simulink model "sixDOF_SIM"  (R2015a)
settings: Solver=ode45  StartTime=0.0  StopTime=t_total  MaxStep=60  RelTol=1e-3
values from neighbouring files (symbols this model uses):
  A0 = zeros(3,3)    [PS2.m]    (also in PS3.m = getDCM(triad1, triad2); PS4.m = getDCM(triad1, triad2); PS5.m = getDCM(triad1, triad2); PS7.m = getDCM(triad1, triad2))
  a0 = 6776    [PS1.m]    (also in PS4.m; PS5.m; PS7.m)
  B = Cd*A/M    (= 0)    [PS1.m]    (also in PS4.m; fullStateController.m = eye(7); getQuat_dot.m = [0 w(3) -w(2) w(1); -w(3) 0 w(1) w(2); w(2) -w(1) 0 w(3);   ; linearEuler.m = (dt * B_))
  bGravGrad = 1    [PS1.m]    (also in PS4.m; PS5.m; PS7.m; PS8.m)
  e0 = 0.0004758    [PS1.m]    (also in PS4.m; PS5.m; PS7.m)
  H = 10    [PS1.m]    (also in PS4.m; getRho.m)
  h0 = Re    (= 6371)    [PS1.m]    (also in PS4.m; getRho.m = 6378.137)
  I_principle = S_top.tauCM_P    [PS2.m]    (also in PS3.m; PS4.m; PS5.m; PS7.m)
  incl0 = 51.6397    [PS1.m]    (also in PS4.m = 0; PS5.m = 0; PS7.m = 0)
  J2 = 0    [PS1.m]    (also in PS4.m; PS5.m; PS7.m)
  M0 = [0 0 0]'    [PS2.m]    (also in PS3.m; PS4.m; PS5.m; PS7.m)
  mu = 3.986e14 / 1000^3    (= 398600)    [PS1.m]    (also in PS4.m; PS5.m; PS7.m)
  nu0 = 0    [PS1.m]    (also in PS4.m; PS5.m; PS7.m)
  OMEGA0 = 106.0758    [PS1.m]    (also in PS4.m = 0; PS5.m = 0; PS7.m = 0)
  omega0 = 233.6745    [PS1.m]    (also in PS4.m = 0; PS5.m = 0; PS7.m = 0)
  Re = 6371    [PS1.m]    (also in PS4.m; PS5.m; PS7.m)
  rho0 = 1.225*1000^3    (= 1225000000)    [PS1.m]    (also in PS4.m; PS5.m; PS7.m; getRho.m)
  w0 = w0_28    [PS2.m]    (also in PS3.m = [0; 0; 10/180*pi*rand()]; PS4.m = w0 + 0.0007*[1 1 1]'; PS5.m = [0 -n0 0]'; PS7.m = [0 -2 0]')
  wEarth0 = [0 0 7.292116e-5]'    [PS1.m]    (also in PS4.m)
settings Model: Creator=Toby  LastModifiedBy=Toby
settings DataIOCC: SaveTime=off

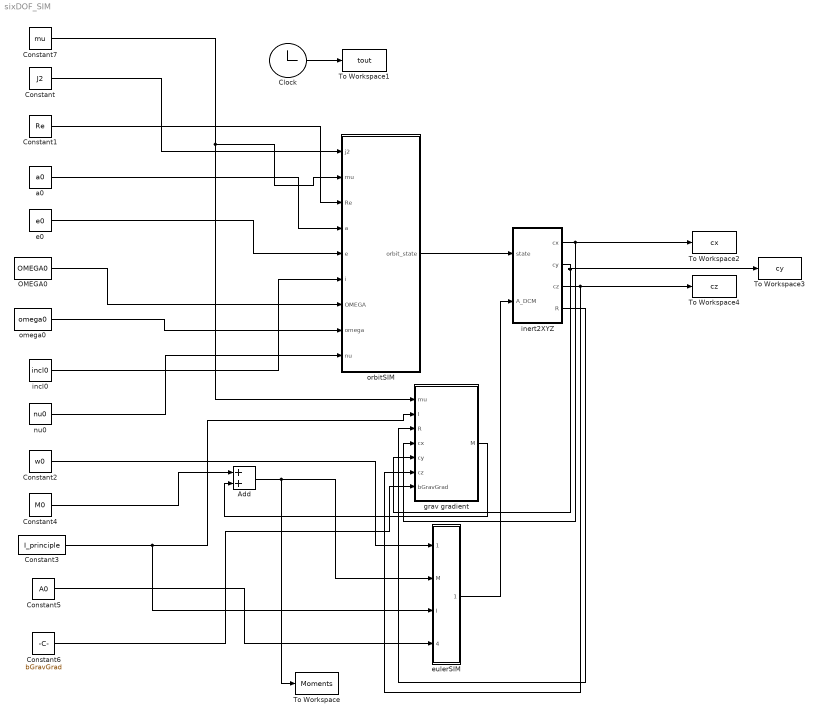
== system sixDOF_SIM ==
  Add : Sum
  Clock : Clock
  Constant : Constant  Value=J2
  Constant1 : Constant  Value=Re
  Constant2 : Constant  Value=w0
  Constant3 : Constant  Value=I_principle
  Constant4 : Constant  Value=M0
  Constant5 : Constant  Value=A0
  Constant6 : Constant  Value=bGravGrad
  Constant7 : Constant  Value=mu
  OMEGA0 : Constant  Value=OMEGA0
  To Workspace : ToWorkspace  VariableName=Moments  SampleTime=-1
  To Workspace1 : ToWorkspace  VariableName=tout  SampleTime=-1
  To Workspace2 : ToWorkspace  VariableName=cx  SampleTime=-1
  To Workspace3 : ToWorkspace  VariableName=cy  SampleTime=-1
  To Workspace4 : ToWorkspace  VariableName=cz  SampleTime=-1
  a0 : Constant  Value=a0
  e0 : Constant  Value=e0
  eulerSIM : Subsystem
  grav gradient : MATLAB Function  TreatAsAtomicUnit=on
  incl0 : Constant  Value=incl0
  inert2XYZ : MATLAB Function  TreatAsAtomicUnit=on
  nu0 : Constant  Value=nu0
  omega0 : Constant  Value=omega0
  orbitSIM : Subsystem
  wires:
  Clock/1 -> To Workspace1/1
  Constant7/1 -> grav gradient/1(mu), orbitSIM/2(mu)
  Constant/1 -> orbitSIM/1(j2)
  Constant1/1 -> orbitSIM/3(Re)
  a0/1 -> orbitSIM/4(a)
  e0/1 -> orbitSIM/5(e)
  OMEGA0/1 -> orbitSIM/7(OMEGA)
  omega0/1 -> orbitSIM/8(omega)
  incl0/1 -> orbitSIM/6(i)
  nu0/1 -> orbitSIM/9(nu)
  Add/1 -> To Workspace/1, eulerSIM/2(M)
  Constant2/1 -> eulerSIM/1(w0)
  Constant3/1 -> grav gradient/2(I), eulerSIM/3(I)
  Constant4/1 -> Add/1
  Constant5/1 -> eulerSIM/4(A0)
  grav gradient/1(M) -> Add/2
  orbitSIM/1(orbit_state) -> inert2XYZ/1(state)
  inert2XYZ/1(cx) -> grav gradient/4(cx), To Workspace2/1
  inert2XYZ/2(cy) -> To Workspace3/1, grav gradient/5(cy)
  inert2XYZ/4(R) -> grav gradient/3(R)
  inert2XYZ/3(cz) -> To Workspace4/1, grav gradient/6(cz)
  eulerSIM/1(A_DCM) -> inert2XYZ/2(A_DCM)
  Constant6/1 -> grav gradient/7(bGravGrad)

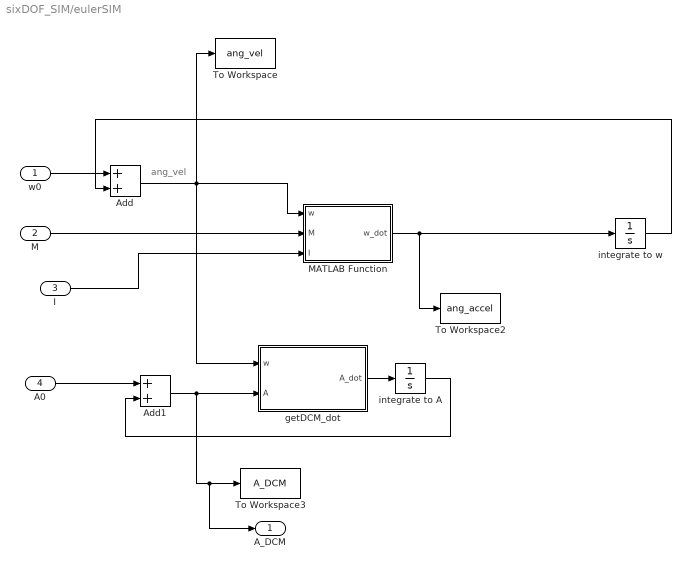
== system sixDOF_SIM/eulerSIM ==
  note: ang_vel
  w0 : Inport
  M : Inport  Port=2
  I : Inport  Port=3
  A0 : Inport  Port=4
  Add : Sum
  Add1 : Sum
  MATLAB Function : MATLAB Function  TreatAsAtomicUnit=on
  To Workspace : ToWorkspace  VariableName=ang_vel  SampleTime=-1
  To Workspace2 : ToWorkspace  VariableName=ang_accel  SampleTime=-1
  To Workspace3 : ToWorkspace  VariableName=A_DCM  SampleTime=-1
  getDCM_dot : MATLAB Function  TreatAsAtomicUnit=on
  integrate to A : Integrator
  integrate to w : Integrator
  A_DCM : Outport
  wires:
  w0/1 -> Add/1
  M/1 -> MATLAB Function/2(M)
  Add1/1 -> A_DCM/1, To Workspace3/1, getDCM_dot/2(A)
  I/1 -> MATLAB Function/3(I)
  getDCM_dot/1(A_dot) -> integrate to A/1
  A0/1 -> Add1/1
  integrate to A/1 -> Add1/2
  MATLAB Function/1(w_dot) -> integrate to w/1, To Workspace2/1
  integrate to w/1 -> Add/2
  Add/1 -> getDCM_dot/1(w), To Workspace/1, MATLAB Function/1(w)

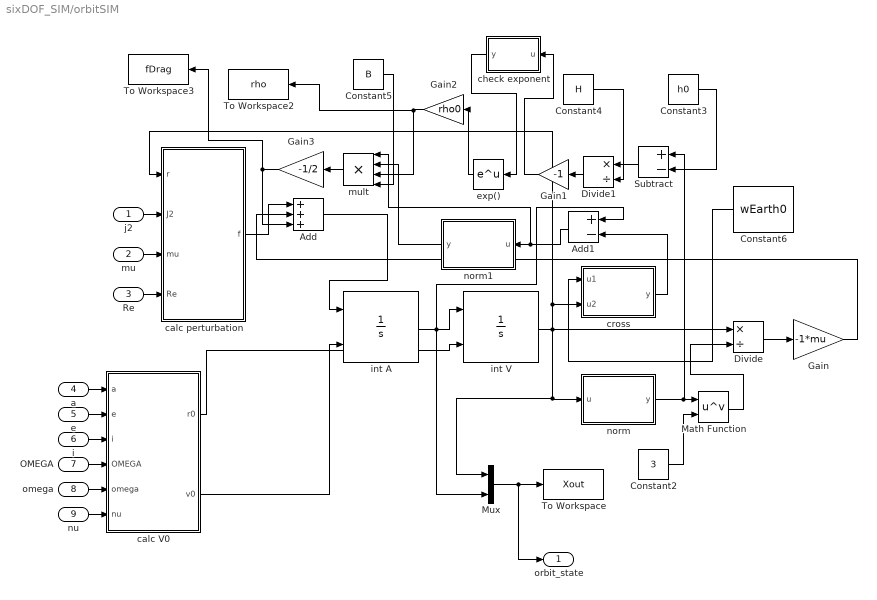
== system sixDOF_SIM/orbitSIM ==
  j2 : Inport
  mu : Inport  Port=2
  Re : Inport  Port=3
  a : Inport  Port=4
  e : Inport  Port=5
  i : Inport  Port=6
  OMEGA : Inport  Port=7
  omega : Inport  Port=8
  nu : Inport  Port=9
  Add : Sum  Inputs=+++
  Add1 : Sum  Inputs=+-
  Constant2 : Constant  Value=3
  Constant3 : Constant  Value=h0
  Constant4 : Constant  Value=H
  Constant5 : Constant  Value=B
  Constant6 : Constant  Value=wEarth0
  Divide : Product  Inputs=*/
  Divide1 : Product  Inputs=*/
  Gain : Gain  Gain=-1*mu
  Gain1 : Gain  Gain=-1
  Gain2 : Gain  Gain=rho0
  Gain3 : Gain  Gain=-1/2
  Math Function : Math  Operator=pow  SaturateOnIntegerOverflow=on
  Mux : Mux  Inputs=2
  Subtract : Sum  Inputs=+-
  To Workspace : ToWorkspace  VariableName=Xout  SampleTime=-1
  To Workspace2 : ToWorkspace  VariableName=rho  SampleTime=-1
  To Workspace3 : ToWorkspace  VariableName=fDrag  SampleTime=-1
  calc V0 : MATLAB Function  TreatAsAtomicUnit=on
  calc perturbation : MATLAB Function  TreatAsAtomicUnit=on
  check exponent : MATLAB Function  TreatAsAtomicUnit=on
  cross : MATLAB Function  TreatAsAtomicUnit=on
  exp() : Math  SaturateOnIntegerOverflow=on
  int A : Integrator  InitialConditionSource=external
  int V : Integrator  InitialConditionSource=external
  mult : Product  Inputs=****
  norm : MATLAB Function  TreatAsAtomicUnit=on
  norm1 : MATLAB Function  TreatAsAtomicUnit=on
  orbit_state : Outport
  wires:
  calc V0/1(r0) -> int V/2
  Divide1/1 -> Gain1/1
  Constant3/1 -> Subtract/2
  Add/1 -> int A/1
  Mux/1 -> orbit_state/1, To Workspace/1
  norm/1(y) -> Subtract/1, Math Function/1
  Constant5/1 -> mult/4
  int V/1 -> calc perturbation/1(r), cross/2(u2), norm/1(u), Mux/1, Divide/1
  Math Function/1 -> Divide/2
  Divide/1 -> Gain/1
  Gain/1 -> Add/2
  Constant4/1 -> Divide1/2
  cross/1(y) -> Add1/2
  check exponent/1(y) -> exp()/1
  calc V0/2(v0) -> int A/2
  int A/1 -> Add1/1, Mux/2, int V/1
  mult/1 -> Gain3/1
  exp()/1 -> Gain2/1
  Subtract/1 -> Divide1/1
  Constant6/1 -> cross/1(u1)
  Add1/1 -> mult/1, norm1/1(u)
  Gain3/1 -> To Workspace3/1, Add/3
  norm1/1(y) -> mult/2
  Gain1/1 -> check exponent/1(u)
  Gain2/1 -> To Workspace2/1, mult/3
  calc perturbation/1(f) -> Add/1
  Constant2/1 -> Math Function/2
  e/1 -> calc V0/2(e)
  i/1 -> calc V0/3(i)
  OMEGA/1 -> calc V0/4(OMEGA)
  a/1 -> calc V0/1(a)
  Re/1 -> calc perturbation/4(Re)
  mu/1 -> calc perturbation/3(mu)
  omega/1 -> calc V0/5(omega)
  j2/1 -> calc perturbation/2(J2)
  nu/1 -> calc V0/6(nu)

== matlab function sixDOF_SIM/orbitSIM/norm ==
  data: u input; y output
function y = fcn(u)
%#codegen

y = norm(u);

== matlab function sixDOF_SIM/orbitSIM/calc perturbation ==
  data: r input; f output; J2 input; mu input; Re input
function f = fcn(r, J2, mu, Re)
% NOTE! EVERYTHING IN DEGREES
% 
% fR = -3*mu*J2*Re^2/(2*r^4)*(1-3*sind(incl)^2*sind(u)^2);
% fT = -3*mu*J2*Re^2/(2*r^4)*(sind(incl)^2*sind(u)*cosd(u));
% fN = -3*mu*J2*Re^2/(2*r^4)*(sind(incl)*cosd(incl)*sind(u));
rMag = norm(r);
rDir = r ./ norm(r);
f = -mu*J2*Re^2/2*( [0, 0, 6*r(3)/rMag^5]' + ...
      (3/rMag^4 - 15*(r(3)^2/rMag^6)).*rDir);

end

== matlab function sixDOF_SIM/orbitSIM/calc V0 ==
  data: a input; r0 output; e input; i input; OMEGA input; omega input; nu input; v0 output
function [r0, v0] = fcn(a, e, i, OMEGA, omega, nu)
%#codegen
[r0, v0] = OE2XV(a, e, i, OMEGA, omega, nu);
end

== matlab function sixDOF_SIM/orbitSIM/norm1 ==
  data: u input; y output
function y = fcn(u)
%#codegen

y = norm(u);

== matlab function sixDOF_SIM/orbitSIM/cross ==
  data: u1 input; y output; u2 input
function y = fcn(u1,u2)
%#codegen

y = cross(u1,u2);

== matlab function sixDOF_SIM/orbitSIM/check exponent ==
  data: u input; y output
function y = fcn(u)
%#codegen
if u>0
  y = 0;
else
  y = u;
end

== matlab function sixDOF_SIM/eulerSIM/MATLAB Function ==
  data: w input; w_dot output; M input; I input
function w_dot = eulerRHS(w, M, I)
% principle axis euler eq
% w is 3x1 rotational velocity
% M is 3x1 external torques
Ix = I(1,1); Iy = I(2,2); Iz = I(3,3);
w_dot = zeros(3,1);
w_dot(1) = (M(1) - (Iz - Iy)*w(2)*w(3) ) / Ix;
w_dot(2) = (M(2) - (Ix - Iz)*w(1)*w(3) ) / Iy;
w_dot(3) = (M(3) - (Iy - Ix)*w(1)*w(2) ) / Iz;
end

== matlab function sixDOF_SIM/eulerSIM/getDCM_dot ==
  data: w input; A_dot output; A input
function A_dot   = getDCM_dot( w, A )
%GETDCM_DOT calculate time-derivative of DCM
% w is ang vel of body axes w.r.t. inertial EXPRESSED IN INERTIAL
[ A_dot ] = getDCM_dot( w, A );

end

== matlab function sixDOF_SIM/grav gradient ==
  data: mu input; M output; I input; R input; cx input; cy input; cz input; bGravGrad input
function M = fcn(mu, I, R, cx, cy, cz, bGravGrad)
%#codegen
if bGravGrad
  M = gravGradient( mu, I, R, cx, cy, cz );
else
  M = [0 0 0]';
end

== matlab function sixDOF_SIM/inert2XYZ ==
  data: cx output; state input; A_DCM input; cy output; cz output; R output
function [cx, cy, cz, R] = fcn(state, A_DCM)
%#codegen
%A should be principle to inertial
A = getP2IfromA_DCM( A_DCM );
R = norm(state(1:3));
c = 1 / R * A' * state(1:3);
cx = c(1);
cy = c(2);
cz = c(3);
